simulink model "ControlePD_5juntas_G"  (R2020a)
settings: Solver=FixedStepAuto  StartTime=0.0  StopTime=10  FixedStep=Ts
values from neighbouring files (symbols this model uses):
  Beff = 50    [controle_FF.m]    (also in controle_PD.m)
  ganho_degrau = [5;5;5;5;5]    [controle_PD.m]
  Jeff = 0.5    [controle_FF.m]    (also in controle_PD.m)
  K = (90/12)*(2*pi/60)    (= 0.785398163397)    [controle_FF.m]    (also in controle_PD.m)
  Kd = (2*xi*wn*Jeff - Beff)/K    (= -44.5633840657)    [controle_FF.m]    (also in controle_PD.m)
  Kp = (wn^2*Jeff)/K    (= 143.239448783)    [controle_FF.m]    (also in controle_PD.m)
  N = 3    [controle_FF.m]    (also in controle_PD.m)
  r = 1./[231.22*4 139.138 139.138 231.22 231.22]    [controle_FF.m]    (also in controle_PD.m)
  SP_theta = [0 0 0 0 0]    [controle_FF.m]    (also in controle_PD.m = [0;0;0;0;0])
  tempo_degrau = [10;20;30;40;50]    [controle_PD.m]
libraries: simulink_extras x20
(part 1 of 3)
settings Model: Creator=Karoline  LastModifiedBy=lunet
settings DataIOCC: ReturnWorkspaceOutputs=off
settings DebuggingCC: ArithmeticOperatorsInVariantConditions=warning
settings SFSimCC: SimUseLocalCustomCode=off  CustomCodeUndefinedFunction=UseInterfaceOnly
settings RTWCC: RTWUseLocalCustomCode=off
settings CodeAppCC: StateflowObjectComments=on

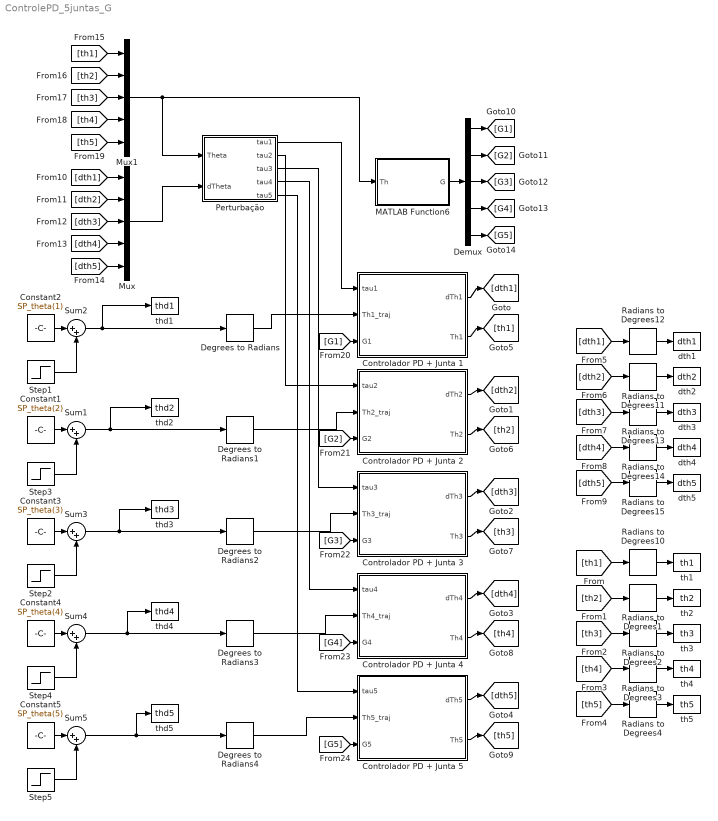
== system ControlePD_5juntas_G ==
  Constant1 : Constant  Value=SP_theta(2)
  Constant2 : Constant  Value=SP_theta(1)
  Constant3 : Constant  Value=SP_theta(3)
  Constant4 : Constant  Value=SP_theta(4)
  Constant5 : Constant  Value=SP_theta(5)
  Controlador PD + Junta 1 : Subsystem
  Controlador PD + Junta 2 : Subsystem
  Controlador PD + Junta 3 : Subsystem
  Controlador PD + Junta 4 : Subsystem
  Controlador PD + Junta 5 : Subsystem
  Degrees to Radians{,1..4} (5 alike) : simulink_extras/Transformations/Degrees to Radians
  Demux : Demux  Outputs=5
  MATLAB Function6 : MATLAB Function  TreatAsAtomicUnit=on
  Mux : Mux  Inputs=5
  Mux1 : Mux  Inputs=5
  Perturbação : Subsystem
  Radians to Degrees{1..4,10..15} (10 alike) : simulink_extras/Transformations/Radians to Degrees
  Step1 : Step  Time=tempo_degrau(1)  After=ganho_degrau(1)  SampleTime=0
  Step2 : Step  Time=tempo_degrau(3)  After=ganho_degrau(3)  SampleTime=0
  Step3 : Step  Time=tempo_degrau(2)  After=ganho_degrau(2)  SampleTime=0
  Step4 : Step  Time=tempo_degrau(4)  After=ganho_degrau(4)  SampleTime=0
  Step5 : Step  Time=tempo_degrau(5)  After=ganho_degrau(5)  SampleTime=0
  Sum{1..5} (5 alike) : Sum  Inputs=|++
  dth1 : ToWorkspace  VariableName=dth1  SampleTime=-1
  dth2 : ToWorkspace  VariableName=dth2  SampleTime=-1
  dth3 : ToWorkspace  VariableName=dth3  SampleTime=-1
  dth4 : ToWorkspace  VariableName=dth4  SampleTime=-1
  dth5 : ToWorkspace  VariableName=dth5  SampleTime=-1
  th1 : ToWorkspace  VariableName=th1  SampleTime=-1
  th2 : ToWorkspace  VariableName=th2  SampleTime=-1
  th3 : ToWorkspace  VariableName=th3  SampleTime=-1
  th4 : ToWorkspace  VariableName=th4  SampleTime=-1
  th5 : ToWorkspace  VariableName=th5  SampleTime=-1
  thd1 : ToWorkspace  VariableName=thd1  SampleTime=-1
  "thd2 " : ToWorkspace  VariableName=thd2  SampleTime=-1
  thd3 : ToWorkspace  VariableName=thd3  SampleTime=-1
  thd4 : ToWorkspace  VariableName=thd4  SampleTime=-1
  thd5 : ToWorkspace  VariableName=thd5  SampleTime=-1
  wires:
  Sum2/1 -> Degrees to Radians/1, thd1/1
  Mux/1 -> Perturbação/2(dTheta)
  Sum3/1 -> Degrees to Radians2/1, thd3/1
  Step3/1 -> Sum1/2
  Sum1/1 -> Degrees to Radians1/1, "thd2 "/1
  Constant1/1 -> Sum1/1
  Degrees to Radians/1 -> Controlador PD + Junta 1/2(Th1_traj)
  Degrees to Radians1/1 -> Controlador PD + Junta 2/2(Th2_traj)
  Degrees to Radians2/1 -> Controlador PD + Junta 3/2(Th3_traj)
  Step1/1 -> Sum2/2
  Constant2/1 -> Sum2/1
  Step2/1 -> Sum3/2
  Constant3/1 -> Sum3/1
  Perturbação/1(tau1) -> Controlador PD + Junta 1/1(tau1)
  Perturbação/2(tau2) -> Controlador PD + Junta 2/1(tau2)
  Perturbação/3(tau3) -> Controlador PD + Junta 3/1(tau3)
  Degrees to Radians4/1 -> Controlador PD + Junta 5/2(Th5_traj)
  Degrees to Radians3/1 -> Controlador PD + Junta 4/2(Th4_traj)
  Constant4/1 -> Sum4/1
  Step4/1 -> Sum4/2
  Constant5/1 -> Sum5/1
  Step5/1 -> Sum5/2
  Sum5/1 -> Degrees to Radians4/1, thd5/1
  Sum4/1 -> Degrees to Radians3/1, thd4/1
  Perturbação/4(tau4) -> Controlador PD + Junta 4/1(tau4)
  Perturbação/5(tau5) -> Controlador PD + Junta 5/1(tau5)
  [th1] -> Radians to Degrees10/1
  Radians to Degrees10/1 -> th1/1
  [th2] -> Radians to Degrees1/1
  Radians to Degrees1/1 -> th2/1
  [th3] -> Radians to Degrees2/1
  Radians to Degrees2/1 -> th3/1
  [th4] -> Radians to Degrees3/1
  Radians to Degrees3/1 -> th4/1
  [th5] -> Radians to Degrees4/1
  Radians to Degrees4/1 -> th5/1
  [dth1] -> Radians to Degrees12/1
  [dth4] -> Radians to Degrees14/1
  Radians to Degrees12/1 -> dth1/1
  Radians to Degrees15/1 -> dth5/1
  [dth3] -> Radians to Degrees13/1
  [dth5] -> Radians to Degrees15/1
  Radians to Degrees13/1 -> dth3/1
  [dth2] -> Radians to Degrees11/1
  Radians to Degrees14/1 -> dth4/1
  Radians to Degrees11/1 -> dth2/1
  Controlador PD + Junta 1/1("dTh1 ") -> [dth1]
  Controlador PD + Junta 2/1("dTh2 ") -> [dth2]
  Controlador PD + Junta 3/1("dTh3 ") -> [dth3]
  Controlador PD + Junta 4/1("dTh4 ") -> [dth4]
  Controlador PD + Junta 5/1("dTh5 ") -> [dth5]
  Controlador PD + Junta 1/2(Th1) -> [th1]
  Controlador PD + Junta 2/2(Th2) -> [th2]
  Controlador PD + Junta 3/2(Th3) -> [th3]
  Controlador PD + Junta 4/2(Th4) -> [th4]
  Controlador PD + Junta 5/2(Th5) -> [th5]
  [dth1] -> Mux/1
  [dth2] -> Mux/2
  [dth3] -> Mux/3
  [dth4] -> Mux/4
  [dth5] -> Mux/5
  [th1] -> Mux1/1
  [th4] -> Mux1/4
  [th5] -> Mux1/5
  [th3] -> Mux1/3
  [th2] -> Mux1/2
  Mux1/1 -> Perturbação/1(Theta), MATLAB Function6/1(Th)
  MATLAB Function6/1(G) -> Demux/1
  [G1] -> Controlador PD + Junta 1/3(G1)
  [G2] -> Controlador PD + Junta 2/3(G2)
  [G3] -> Controlador PD + Junta 3/3(G3)
  [G4] -> Controlador PD + Junta 4/3(G4)
  [G5] -> Controlador PD + Junta 5/3(G5)
  Demux/1 -> [G1]
  Demux/2 -> [G2]
  Demux/5 -> [G5]
  Demux/4 -> [G4]
  Demux/3 -> [G3]

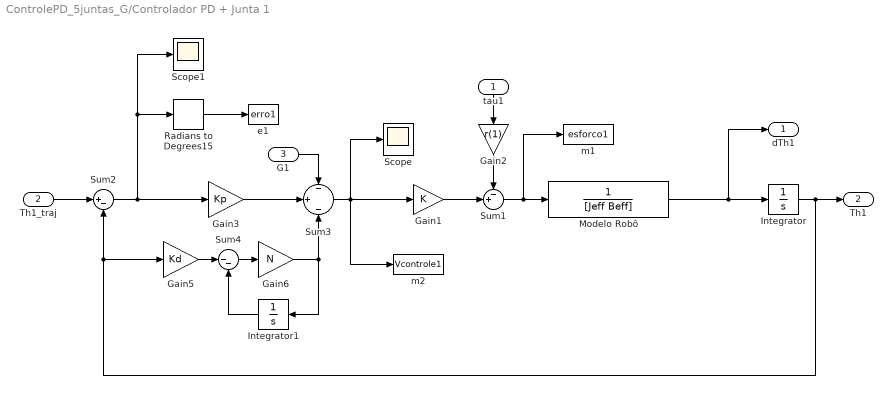
== system ControlePD_5juntas_G/Controlador PD + Junta 1 ==
  tau1 : Inport
  Th1_traj : Inport  Port=2
  G1 : Inport  Port=3
  Gain1 : Gain  Gain=K
  Gain2 : Gain  Gain=r(1)
  Gain3 : Gain  Gain=Kp
  Gain5 : Gain  Gain=Kd
  Gain6 : Gain  Gain=N
  Integrator : Integrator  InitialCondition=SP_theta(1)*pi/180
  Integrator1 : Integrator
  Modelo Robô : TransferFcn  Denominator=[Jeff Beff]
  Radians to Degrees15 : simulink_extras/Transformations/Radians to Degrees
  Scope : Scope
  Scope1 : Scope
  Sum1 : Sum  Inputs=-+|
  Sum2 : Sum  Inputs=|+-
  Sum3 : Sum  Inputs=-|+|-
  Sum4 : Sum  Inputs=|--
  e1 : ToWorkspace  VariableName=erro1  SampleTime=-1
  m1 : ToWorkspace  VariableName=esforco1  SampleTime=-1
  m2 : ToWorkspace  VariableName=Vcontrole1  SampleTime=-1
  "dTh1 " : Outport  VectorParamsAs1DForOutWhenUnconnected=off
  Th1 : Outport  Port=2  VectorParamsAs1DForOutWhenUnconnected=off
  wires:
  tau1/1 -> Gain2/1
  Gain1/1 -> Sum1/2
  Sum1/1 -> m1/1, Modelo Robô/1
  Th1_traj/1 -> Sum2/1
  Gain2/1 -> Sum1/1
  Radians to Degrees15/1 -> e1/1
  Gain3/1 -> Sum3/2
  Sum3/1 -> m2/1, Scope/1, Gain1/1
  Modelo Robô/1 -> Integrator/1, "dTh1 "/1
  Sum4/1 -> Gain6/1
  Integrator1/1 -> Sum4/2
  Gain5/1 -> Sum4/1
  Gain6/1 -> Sum3/3, Integrator1/1
  Sum2/1 -> Gain3/1, Radians to Degrees15/1, Scope1/1
  Integrator/1 -> Th1/1, Gain5/1, Sum2/2
  G1/1 -> Sum3/1

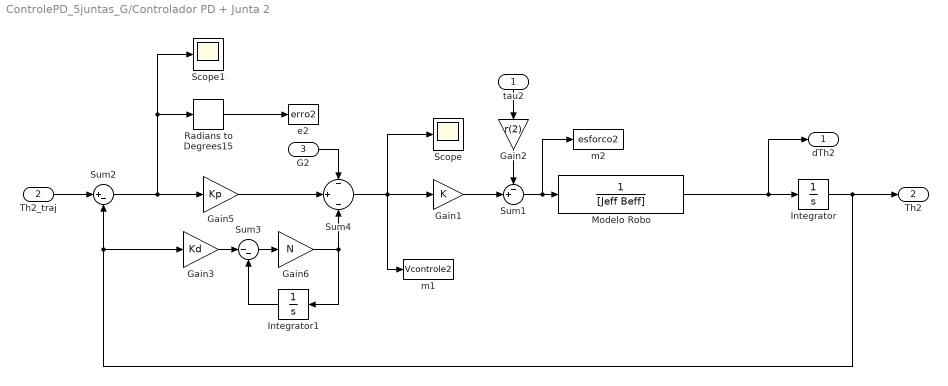
== system ControlePD_5juntas_G/Controlador PD + Junta 2 ==
  tau2 : Inport
  Th2_traj : Inport  Port=2
  G2 : Inport  Port=3
  Gain1 : Gain  Gain=K
  Gain2 : Gain  Gain=r(2)
  Gain3 : Gain  Gain=Kd
  Gain5 : Gain  Gain=Kp
  Gain6 : Gain  Gain=N
  Integrator : Integrator  InitialCondition=SP_theta(2)*pi/180
  Integrator1 : Integrator
  "Modelo Robo " : TransferFcn  Denominator=[Jeff Beff]
  Radians to Degrees15 : simulink_extras/Transformations/Radians to Degrees
  Scope : Scope
  Scope1 : Scope
  Sum1 : Sum  Inputs=-+|
  Sum2 : Sum  Inputs=|+-
  Sum3 : Sum  Inputs=|--
  Sum4 : Sum  Inputs=-|+|-
  e2 : ToWorkspace  VariableName=erro2  SampleTime=-1
  m1 : ToWorkspace  VariableName=Vcontrole2  SampleTime=-1
  m2 : ToWorkspace  VariableName=esforco2  SampleTime=-1
  "dTh2 " : Outport  VectorParamsAs1DForOutWhenUnconnected=off
  Th2 : Outport  Port=2  VectorParamsAs1DForOutWhenUnconnected=off
  wires:
  tau2/1 -> Gain2/1
  Gain1/1 -> Sum1/2
  Sum1/1 -> m2/1, "Modelo Robo "/1
  Th2_traj/1 -> Sum2/1
  Gain2/1 -> Sum1/1
  Radians to Degrees15/1 -> e2/1
  Gain5/1 -> Sum4/2
  Sum4/1 -> m1/1, Scope/1, Gain1/1
  Integrator/1 -> Th2/1, Gain3/1, Sum2/2
  "Modelo Robo "/1 -> "dTh2 "/1, Integrator/1
  Gain6/1 -> Sum4/3, Integrator1/1
  Integrator1/1 -> Sum3/2
  Sum3/1 -> Gain6/1
  Gain3/1 -> Sum3/1
  Sum2/1 -> Radians to Degrees15/1, Scope1/1, Gain5/1
  G2/1 -> Sum4/1

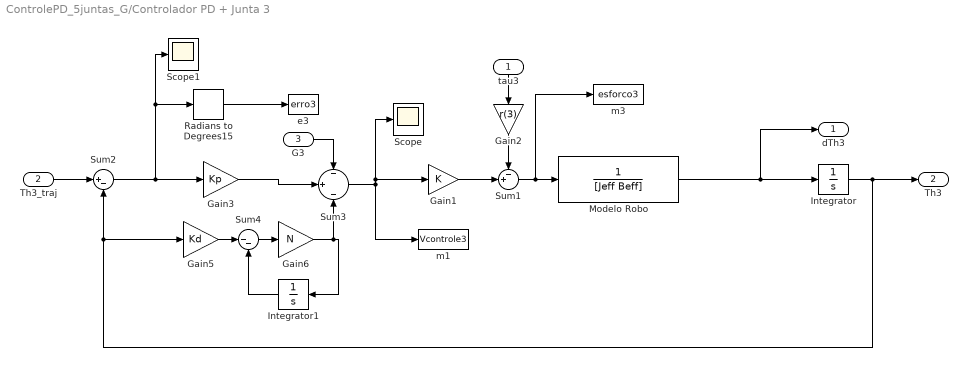
== system ControlePD_5juntas_G/Controlador PD + Junta 3 ==
  tau3 : Inport
  Th3_traj : Inport  Port=2
  G3 : Inport  Port=3
  Gain1 : Gain  Gain=K
  Gain2 : Gain  Gain=r(3)
  Gain3 : Gain  Gain=Kp
  Gain5 : Gain  Gain=Kd
  Gain6 : Gain  Gain=N
  Integrator : Integrator  InitialCondition=SP_theta(3)*pi/180
  Integrator1 : Integrator
  Modelo Robo : TransferFcn  Denominator=[Jeff Beff]
  Radians to Degrees15 : simulink_extras/Transformations/Radians to Degrees
  Scope : Scope
  Scope1 : Scope
  Sum1 : Sum  Inputs=-+|
  Sum2 : Sum  Inputs=|+-
  Sum3 : Sum  Inputs=-|+|-
  Sum4 : Sum  Inputs=|--
  e3 : ToWorkspace  VariableName=erro3  SampleTime=-1
  m1 : ToWorkspace  VariableName=Vcontrole3  SampleTime=-1
  m3 : ToWorkspace  VariableName=esforco3  SampleTime=-1
  "dTh3 " : Outport  VectorParamsAs1DForOutWhenUnconnected=off
  Th3 : Outport  Port=2  VectorParamsAs1DForOutWhenUnconnected=off
  wires:
  tau3/1 -> Gain2/1
  Gain1/1 -> Sum1/2
  Sum1/1 -> m3/1, Modelo Robo/1
  Th3_traj/1 -> Sum2/1
  Gain2/1 -> Sum1/1
  Radians to Degrees15/1 -> e3/1
  Gain3/1 -> Sum3/2
  Sum3/1 -> Scope/1, Gain1/1, m1/1
  Integrator/1 -> Th3/1, Gain5/1, Sum2/2
  Modelo Robo/1 -> Integrator/1, "dTh3 "/1
  Gain6/1 -> Integrator1/1, Sum3/3
  Integrator1/1 -> Sum4/2
  Sum4/1 -> Gain6/1
  Gain5/1 -> Sum4/1
  Sum2/1 -> Gain3/1, Radians to Degrees15/1, Scope1/1
  G3/1 -> Sum3/1

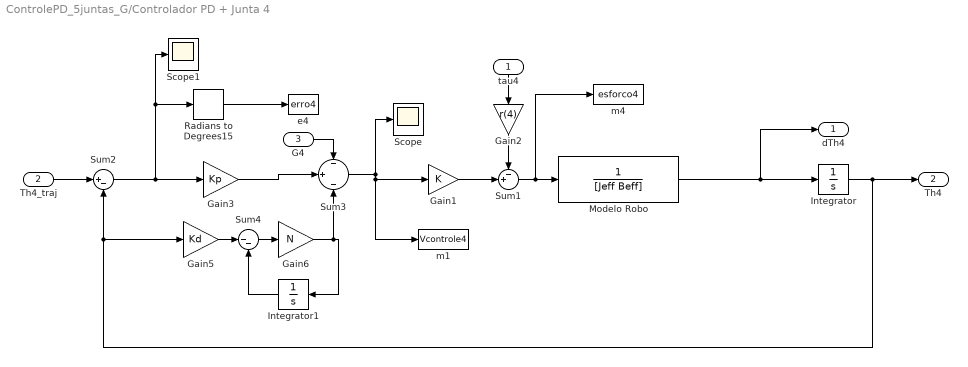
== system ControlePD_5juntas_G/Controlador PD + Junta 4 ==
  tau4 : Inport
  Th4_traj : Inport  Port=2
  G4 : Inport  Port=3
  Gain1 : Gain  Gain=K
  Gain2 : Gain  Gain=r(4)
  Gain3 : Gain  Gain=Kp
  Gain5 : Gain  Gain=Kd
  Gain6 : Gain  Gain=N
  Integrator : Integrator  InitialCondition=SP_theta(4)*pi/180
  Integrator1 : Integrator
  Modelo Robo : TransferFcn  Denominator=[Jeff Beff]
  Radians to Degrees15 : simulink_extras/Transformations/Radians to Degrees
  Scope : Scope
  Scope1 : Scope
  Sum1 : Sum  Inputs=-+|
  Sum2 : Sum  Inputs=|+-
  Sum3 : Sum  Inputs=-|+|-
  Sum4 : Sum  Inputs=|--
  e4 : ToWorkspace  VariableName=erro4  SampleTime=-1
  m1 : ToWorkspace  VariableName=Vcontrole4  SampleTime=-1
  m4 : ToWorkspace  VariableName=esforco4  SampleTime=-1
  "dTh4 " : Outport  VectorParamsAs1DForOutWhenUnconnected=off
  Th4 : Outport  Port=2  VectorParamsAs1DForOutWhenUnconnected=off
  wires:
  tau4/1 -> Gain2/1
  Gain1/1 -> Sum1/2
  Sum1/1 -> m4/1, Modelo Robo/1
  Th4_traj/1 -> Sum2/1
  Gain2/1 -> Sum1/1
  Radians to Degrees15/1 -> e4/1
  Gain3/1 -> Sum3/2
  Sum3/1 -> m1/1, Gain1/1, Scope/1
  Integrator/1 -> Th4/1, Sum2/2, Gain5/1
  Modelo Robo/1 -> Integrator/1, "dTh4 "/1
  Gain6/1 -> Integrator1/1, Sum3/3
  Integrator1/1 -> Sum4/2
  Sum4/1 -> Gain6/1
  Gain5/1 -> Sum4/1
  Sum2/1 -> Gain3/1, Radians to Degrees15/1, Scope1/1
  G4/1 -> Sum3/1

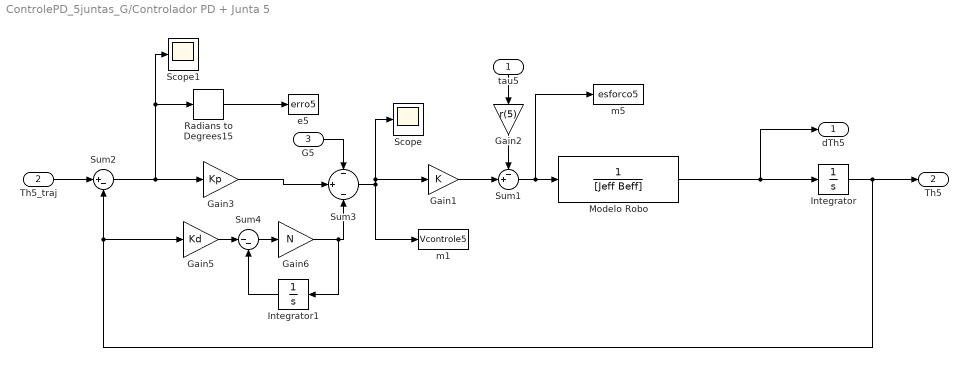
== system ControlePD_5juntas_G/Controlador PD + Junta 5 ==
  tau5 : Inport
  Th5_traj : Inport  Port=2
  G5 : Inport  Port=3
  Gain1 : Gain  Gain=K
  Gain2 : Gain  Gain=r(5)
  Gain3 : Gain  Gain=Kp
  Gain5 : Gain  Gain=Kd
  Gain6 : Gain  Gain=N
  Integrator : Integrator  InitialCondition=SP_theta(5)*pi/180
  Integrator1 : Integrator
  Modelo Robo : TransferFcn  Denominator=[Jeff Beff]
  Radians to Degrees15 : simulink_extras/Transformations/Radians to Degrees
  Scope : Scope
  Scope1 : Scope
  Sum1 : Sum  Inputs=-+|
  Sum2 : Sum  Inputs=|+-
  Sum3 : Sum  Inputs=-|+|-
  Sum4 : Sum  Inputs=|--
  e5 : ToWorkspace  VariableName=erro5  SampleTime=-1
  m1 : ToWorkspace  VariableName=Vcontrole5  SampleTime=-1
  m5 : ToWorkspace  VariableName=esforco5  SampleTime=-1
  "dTh5 " : Outport  VectorParamsAs1DForOutWhenUnconnected=off
  Th5 : Outport  Port=2  VectorParamsAs1DForOutWhenUnconnected=off
  wires:
  tau5/1 -> Gain2/1
  Gain1/1 -> Sum1/2
  Sum1/1 -> m5/1, Modelo Robo/1
  Th5_traj/1 -> Sum2/1
  Gain2/1 -> Sum1/1
  Radians to Degrees15/1 -> e5/1
  Gain3/1 -> Sum3/2
  Sum3/1 -> Scope/1, Gain1/1, m1/1
  Integrator/1 -> Th5/1, Gain5/1, Sum2/2
  Modelo Robo/1 -> Integrator/1, "dTh5 "/1
  Gain6/1 -> Sum3/3, Integrator1/1
  Integrator1/1 -> Sum4/2
  Sum4/1 -> Gain6/1
  Gain5/1 -> Sum4/1
  Sum2/1 -> Gain3/1, Radians to Degrees15/1, Scope1/1
  G5/1 -> Sum3/1

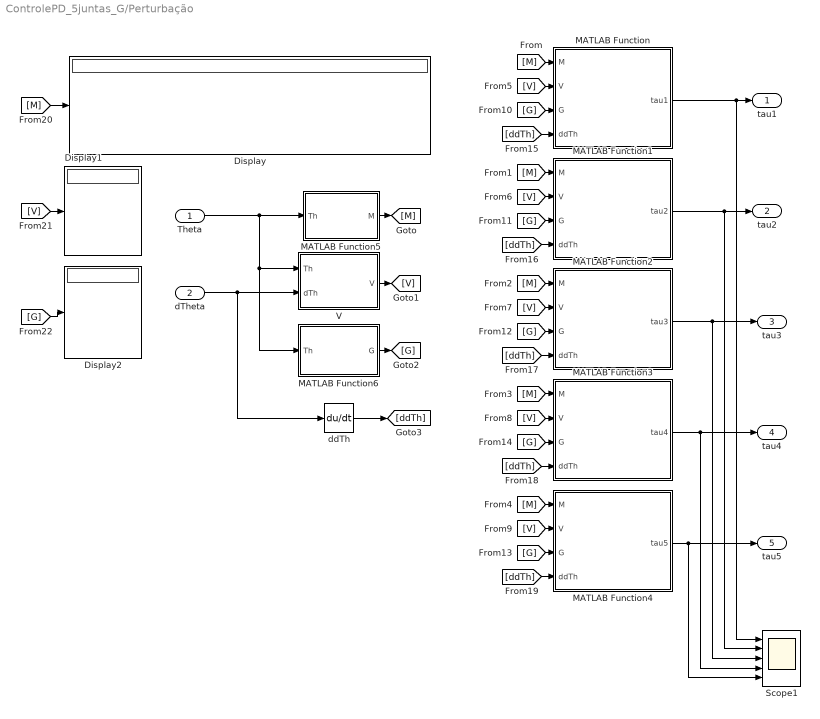
== system ControlePD_5juntas_G/Perturbação ==
  Theta : Inport
  dTheta : Inport  Port=2
  Display : Display
  Display1 : Display
  Display2 : Display
  MATLAB Function : MATLAB Function  TreatAsAtomicUnit=on
  MATLAB Function1 : MATLAB Function  TreatAsAtomicUnit=on
  MATLAB Function2 : MATLAB Function  TreatAsAtomicUnit=on
  MATLAB Function3 : MATLAB Function  TreatAsAtomicUnit=on
  MATLAB Function4 : MATLAB Function  TreatAsAtomicUnit=on
  MATLAB Function5 : MATLAB Function  TreatAsAtomicUnit=on
  MATLAB Function6 : MATLAB Function  TreatAsAtomicUnit=on
  Scope1 : Scope  NumInputPorts=5
  V : MATLAB Function  TreatAsAtomicUnit=on
  ddTh : Derivative
  tau1 : Outport  VectorParamsAs1DForOutWhenUnconnected=off
  tau2 : Outport  Port=2  VectorParamsAs1DForOutWhenUnconnected=off
  tau3 : Outport  Port=3  VectorParamsAs1DForOutWhenUnconnected=off
  tau4 : Outport  Port=4  VectorParamsAs1DForOutWhenUnconnected=off
  tau5 : Outport  Port=5  VectorParamsAs1DForOutWhenUnconnected=off
  wires:
  dTheta/1 -> V/2(dTh), ddTh/1
  MATLAB Function/1(tau1) -> tau1/1, Scope1/1
  Theta/1 -> MATLAB Function5/1(Th), MATLAB Function6/1(Th), V/1(Th)
  MATLAB Function1/1(tau2) -> tau2/1, Scope1/2
  MATLAB Function2/1(tau3) -> tau3/1, Scope1/3
  MATLAB Function3/1(tau4) -> tau4/1, Scope1/4
  MATLAB Function4/1(tau5) -> tau5/1, Scope1/5
  ddTh/1 -> [ddTh]
  MATLAB Function5/1(M) -> [M]
  V/1(V) -> [V]
  MATLAB Function6/1(G) -> [G]
  [M] -> MATLAB Function/1(M)
  [M] -> MATLAB Function1/1(M)
  [M] -> MATLAB Function2/1(M)
  [M] -> MATLAB Function3/1(M)
  [M] -> MATLAB Function4/1(M)
  [V] -> MATLAB Function/2(V)
  [V] -> MATLAB Function1/2(V)
  [V] -> MATLAB Function2/2(V)
  [V] -> MATLAB Function3/2(V)
  [V] -> MATLAB Function4/2(V)
  [G] -> MATLAB Function/3(G)
  [G] -> MATLAB Function1/3(G)
  [G] -> MATLAB Function2/3(G)
  [G] -> MATLAB Function4/3(G)
  [G] -> MATLAB Function3/3(G)
  [ddTh] -> MATLAB Function/4(ddTh)
  [ddTh] -> MATLAB Function1/4(ddTh)
  [ddTh] -> MATLAB Function2/4(ddTh)
  [ddTh] -> MATLAB Function3/4(ddTh)
  [ddTh] -> MATLAB Function4/4(ddTh)
  [M] -> Display/1
  [V] -> Display1/1
  [G] -> Display2/1

== matlab function ControlePD_5juntas_G/Perturbação/MATLAB Function1 ==
  data: M input; V input; tau2 output; G input; ddTh input
function tau2  = calcul_dk2(M, V, G, ddTh)

tau2 = M(2,1)*ddTh(1) + M(2,3)*ddTh(3) + M(2,4)*ddTh(4) + M(2,5)*ddTh(5) ...
       + V(2) + G(2);

== matlab function ControlePD_5juntas_G/Perturbação/MATLAB Function2 ==
  data: M input; V input; tau3 output; G input; ddTh input
function tau3  = calcul_dk3(M, V, G, ddTh)

tau3 = M(3,1)*ddTh(1) + M(3,2)*ddTh(2) + M(3,4)*ddTh(4) + M(3,5)*ddTh(5) ...
       + V(3) + G(3);

== matlab function ControlePD_5juntas_G/Perturbação/MATLAB Function3 ==
  data: M input; V input; tau4 output; G input; ddTh input
function tau4  = calcul_dk4(M, V, G, ddTh)

tau4 = M(4,1)*ddTh(1) + M(4,2)*ddTh(2) + M(4,3)*ddTh(3) + M(4,5)*ddTh(5) ...
       + V(4) + G(4);

== matlab function ControlePD_5juntas_G/Perturbação/MATLAB Function4 ==
  data: M input; V input; tau5 output; G input; ddTh input
function tau5  = calcul_dk5(M, V, G, ddTh)

tau5 = M(5,1)*ddTh(1) + M(5,2)*ddTh(2) + M(5,3)*ddTh(3) + M(5,4)*ddTh(4) ...
       + V(5) + G(5);

== matlab function ControlePD_5juntas_G/Perturbação/MATLAB Function6 ==
  data: Th input; G output
function G = calcul_G(Th)

g = 9.80665;
th1 = Th(1);
th2 = Th(2);
th3 = Th(3);
th4 = Th(4);
th5 = Th(5);

G = [                                                                                                                                                                                                                                                                                               0;
 -g*((49*cos(th2)*sin(th3))/125 - cos(th2)/2 + (49*cos(th3)*sin(th2))/125 + (3*cos(th2)*cos(th5)*sin(th3))/40 + (3*cos(th3)*cos(th5)*sin(th2))/40 + (3*cos(th2)*cos(th3)*cos(th4)*sin(th5))/40 - (3*cos(th4)*sin(th2)*sin(th3)*sin(th5))/40);
                 -g*((49*cos(th2)*sin(th3))/125 + (49*cos(th3)*sin(th2))/125 + (3*cos(th2)*cos(th5)*sin(th3))/40 + (3*cos(th3)*cos(th5)*sin(th2))/40 + (3*cos(th2)*cos(th3)*cos(th4)*sin(th5))/40 - (3*cos(th4)*sin(th2)*sin(th3)*sin(th5))/40);
                                                                                                                                                                                                                                                (3*g*sin(th4)*sin(th5)*sin(th2 + th3))/40;
                                                                                       -g*((3*cos(th2)*cos(th3)*sin(th5))/40 - (3*sin(th2)*sin(th3)*sin(th5))/40 + (3*cos(th2)*cos(th4)*cos(th5)*sin(th3))/40 + (3*cos(th3)*cos(th4)*cos(th5)*sin(th2))/40)];

== matlab function ControlePD_5juntas_G/Perturbação/MATLAB Function5 ==
  data: Th input; M output
function M = calcul_M(Th)

th1 = Th(1);
th2 = Th(2);
th3 = Th(3);
th4 = Th(4);
th5 = Th(5);

M = [ (87*cos(th2)^2*cos(th5))/2500 + (87*cos(th3)^2*cos(th5))/2500 - (33*cos(th2)^2*sin(th3))/50 + (53231*cos(th2)^2)/62500 + (8453*cos(th3)^2)/31250 - (9*cos(th5)^2)/3200 - (8453*cos(th2)^2*cos(th3)^2)/15625 - (217*cos(th2)^2*cos(th4)^2)/80000 + (9*cos(th2)^2*cos(th5)^2)/3200 - (217*cos(th3)^2*cos(th4)^2)/80000 + (9*cos(th3)^2*cos(th5)^2)/3200 - (87*cos(th2)^2*cos(th3)^2*cos(th5))/1250 - (33*cos(th2)*cos(th3)*sin(th2))/50 + (217*cos(th2)^2*cos(th3)^2*cos(th4)^2)/40000 - (9*cos(th2)^2*cos(th3)^2*cos(th5)^2)/1600 + (9*cos(th2)^2*cos(th4)^2*cos(th5)^2)/3200 + (9*cos(th3)^2*cos(th4)^2*cos(th5)^2)/3200 - (3*cos(th2)^2*cos(th5)*sin(th3))/80 - (9*cos(th2)^2*cos(th3)^2*cos(th4)^2*cos(th5)^2)/1600 - (3*cos(th2)*cos(th3)*cos(th5)*sin(th2))/80 + (8453*cos(th2)*cos(th3)*sin(th2)*sin(th3))/15625 - (87*cos(th2)*cos(th4)*sin(th2)*sin(th5))/2500 - (87*cos(th3)*cos(th4)*sin(th3)*sin(th5))/2500 - (3*cos(th2)^2*cos(th3)*cos(th4)*sin(th5))/80 + (3*cos(th2)*cos(th4)*sin(th2)*sin(th3)*sin(th5))/80 - (217*cos(th2)*cos(th3)*cos(th4)^2*sin(th2)*sin(th3))/40000 + (9*cos(th2)*cos(th3)*cos(th5)^2*sin(th2)*sin(th3))/1600 + (87*cos(th2)*cos(th3)^2*cos(th4)*sin(th2)*sin(th5))/1250 + (87*cos(th2)^2*cos(th3)*cos(th4)*sin(th3)*sin(th5))/1250 + (87*cos(th2)*cos(th3)*cos(th5)*sin(th2)*sin(th3))/1250 - (9*cos(th2)*cos(th4)*cos(th5)*sin(th2)*sin(th5))/1600 - (9*cos(th3)*cos(th4)*cos(th5)*sin(th3)*sin(th5))/1600 + (9*cos(th2)*cos(th3)*cos(th4)^2*cos(th5)^2*sin(th2)*sin(th3))/1600 + (9*cos(th2)*cos(th3)^2*cos(th4)*cos(th5)*sin(th2)*sin(th5))/800 + (9*cos(th2)^2*cos(th3)*cos(th4)*cos(th5)*sin(th3)*sin(th5))/800 + 3793/80000, -(sin(th4)*(1500*sin(th2)*sin(th5) - 217*cos(th2)*cos(th4)*sin(th3) - 217*cos(th3)*cos(th4)*sin(th2) + 1392*cos(th2)*cos(th3)*sin(th5) - 1392*sin(th2)*sin(th3)*sin(th5) + 225*cos(th2)*cos(th3)*cos(th5)*sin(th5) - 225*cos(th5)*sin(th2)*sin(th3)*sin(th5) + 225*cos(th2)*cos(th4)*cos(th5)^2*sin(th3) + 225*cos(th3)*cos(th4)*cos(th5)^2*sin(th2)))/80000, (sin(th4)*(217*cos(th2)*cos(th4)*sin(th3) + 217*cos(th3)*cos(th4)*sin(th2) - 1392*cos(th2)*cos(th3)*sin(th5) + 1392*sin(th2)*sin(th3)*sin(th5) - 225*cos(th2)*cos(th3)*cos(th5)*sin(th5) + 225*cos(th5)*sin(th2)*sin(th3)*sin(th5) - 225*cos(th2)*cos(th4)*cos(th5)^2*sin(th3) - 225*cos(th3)*cos(th4)*cos(th5)^2*sin(th2)))/80000, (489*cos(th2)*cos(th3))/80000 - (489*sin(th2)*sin(th3))/80000 - (3*cos(th2)*cos(th4)*sin(th5))/160 - (9*cos(th2)*cos(th3)*cos(th5)^2)/3200 + (9*cos(th5)^2*sin(th2)*sin(th3))/3200 + (87*cos(th2)*cos(th4)*sin(th3)*sin(th5))/5000 + (87*cos(th3)*cos(th4)*sin(th2)*sin(th5))/5000 + (9*cos(th2)*cos(th4)*cos(th5)*sin(th3)*sin(th5))/3200 + (9*cos(th3)*cos(th4)*cos(th5)*sin(th2)*sin(th5))/3200, (sin(th4)*(353*cos(th2)*sin(th3) + 353*cos(th3)*sin(th2) - 1500*cos(th2)*cos(th5) + 1392*cos(th2)*cos(th5)*sin(th3) + 1392*cos(th3)*cos(th5)*sin(th2)))/80000;
                                                                                                                                                                                                                                                                                                                                                                                                                                                                                                                                                                                                                                                                                                                                                                                                                                                                                                                                                                                                                                                                                                                                                                                                                                                                                                                                                                                                                                                                                                                                                                                            -(sin(th4)*(1500*sin(th2)*sin(th5) - 217*cos(th2)*cos(th4)*sin(th3) - 217*cos(th3)*cos(th4)*sin(th2) + 1392*cos(th2)*cos(th3)*sin(th5) - 1392*sin(th2)*sin(th3)*sin(th5) + 225*cos(th2)*cos(th3)*cos(th5)*sin(th5) - 225*cos(th5)*sin(th2)*sin(th3)*sin(th5) + 225*cos(th2)*cos(th4)*cos(th5)^2*sin(th3) + 225*cos(th3)*cos(th4)*cos(th5)^2*sin(th2)))/80000,                                                                                                                                                                                                                       (87*cos(th5))/2500 - (33*sin(th3))/50 - (3*cos(th5)*sin(th3))/80 + (217*cos(th4)^2)/80000 + (9*cos(th5)^2)/3200 - (9*cos(th4)^2*cos(th5)^2)/3200 - (3*cos(th3)*cos(th4)*sin(th5))/80 + 54781/62500,                                                                                                                                                                                   (87*cos(th5))/2500 - (33*sin(th3))/100 - (3*cos(th5)*sin(th3))/160 + (217*cos(th4)^2)/80000 + (9*cos(th5)^2)/3200 - (9*cos(th4)^2*cos(th5)^2)/3200 - (3*cos(th3)*cos(th4)*sin(th5))/160 + 72749/250000,                                                                                                                                                                                                                                                                                                                                                                                                                     -(3*sin(th4)*sin(th5)*(75*cos(th5) - 500*sin(th3) + 464))/80000,                                                          (353*cos(th4))/80000 - (3*cos(th3)*sin(th5))/160 + (87*cos(th4)*cos(th5))/5000 - (3*cos(th4)*cos(th5)*sin(th3))/160;
                                                                                                                                                                                                                                                                                                                                                                                                                                                                                                                                                                                                                                                                                                                                                                                                                                                                                                                                                                                                                                                                                                                                                                                                                                                                                                                                                                                                                                                                                                                                                                                                                            (sin(th4)*(217*cos(th2)*cos(th4)*sin(th3) + 217*cos(th3)*cos(th4)*sin(th2) - 1392*cos(th2)*cos(th3)*sin(th5) + 1392*sin(th2)*sin(th3)*sin(th5) - 225*cos(th2)*cos(th3)*cos(th5)*sin(th5) + 225*cos(th5)*sin(th2)*sin(th3)*sin(th5) - 225*cos(th2)*cos(th4)*cos(th5)^2*sin(th3) - 225*cos(th3)*cos(th4)*cos(th5)^2*sin(th2)))/80000,                                                                                                                                                                                                                   (87*cos(th5))/2500 - (33*sin(th3))/100 - (3*cos(th5)*sin(th3))/160 + (217*cos(th4)^2)/80000 + (9*cos(th5)^2)/3200 - (9*cos(th4)^2*cos(th5)^2)/3200 - (3*cos(th3)*cos(th4)*sin(th5))/160 + 72749/250000,                                                                                                                                                                                                                                                                                          (87*cos(th5))/2500 + (217*cos(th4)^2)/80000 + (9*cos(th5)^2)/3200 - (9*cos(th4)^2*cos(th5)^2)/3200 + 72749/250000,                                                                                                                                                                                                                                                                                                                                                                                                                                       -(3*sin(th4)*sin(th5)*(75*cos(th5) + 464))/80000,                                                                                                                                                         (cos(th4)*(1392*cos(th5) + 353))/80000;
                                                                                                                                                                                                                                                                                                                                                                                                                                                                                                                                                                                                                                                                                                                                                                                                                                                                                                                                                                                                                                                                                                                                                                                                                                                                                                                                                                                                                                                                                                                                                      (489*cos(th2)*cos(th3))/80000 - (489*sin(th2)*sin(th3))/80000 - (3*cos(th2)*cos(th4)*sin(th5))/160 - (9*cos(th2)*cos(th3)*cos(th5)^2)/3200 + (9*cos(th5)^2*sin(th2)*sin(th3))/3200 + (87*cos(th2)*cos(th4)*sin(th3)*sin(th5))/5000 + (87*cos(th3)*cos(th4)*sin(th2)*sin(th5))/5000 + (9*cos(th2)*cos(th4)*cos(th5)*sin(th3)*sin(th5))/3200 + (9*cos(th3)*cos(th4)*cos(th5)*sin(th2)*sin(th5))/3200,                                                                                                                                                                                                                                                                                                                                                                               -(3*sin(th4)*sin(th5)*(75*cos(th5) - 500*sin(th3) + 464))/80000,                                                                                                                                                                                                                                                                                                                                                                 -(3*sin(th4)*sin(th5)*(75*cos(th5) + 464))/80000,                                                                                                                                                                                                                                                                                                                                                                                                                                                              489/80000 - (9*cos(th5)^2)/3200,                                                                                                                                                                                                    0;
                                                                                                                                                                                                                                                                                                                                                                                                                                                                                                                                                                                                                                                                                                                                                                                                                                                                                                                                                                                                                                                                                                                                                                                                                                                                                                                                                                                                                                                                                                                                                                                                                                                                                                                                                                                                                                                 (sin(th4)*(353*cos(th2)*sin(th3) + 353*cos(th3)*sin(th2) - 1500*cos(th2)*cos(th5) + 1392*cos(th2)*cos(th5)*sin(th3) + 1392*cos(th3)*cos(th5)*sin(th2)))/80000,                                                                                                                                                                                                                                                                                                               (353*cos(th4))/80000 - (3*cos(th3)*sin(th5))/160 + (87*cos(th4)*cos(th5))/5000 - (3*cos(th4)*cos(th5)*sin(th3))/160,                                                                                                                                                                                                                                                                                                                                                                              (cos(th4)*(1392*cos(th5) + 353))/80000,                                                                                                                                                                                                                                                                                                                                                                                                                                                                                               0,                                                                                                                                                                                            353/80000];
